simulink model "ex2"  (R2020a)
settings: Solver=VariableStepAuto  StartTime=0.0  StopTime=10.0  RelTol=1e-3
settings Model: Creator=EREN  LastModifiedBy=EREN

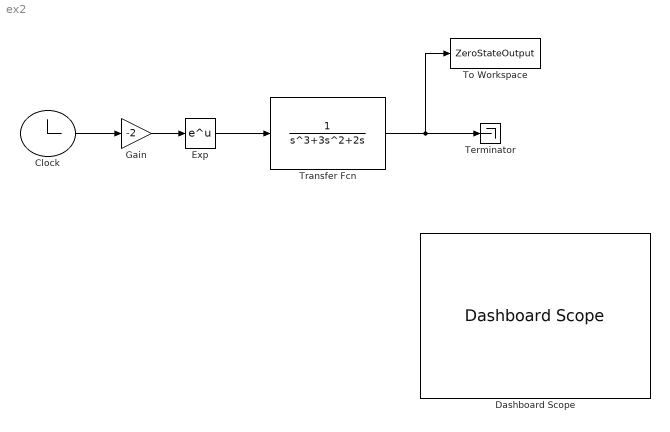
== system ex2 ==
  Clock : Clock
  Dashboard Scope : DashboardScope
  Exp : Math  SaturateOnIntegerOverflow=on
  Gain : Gain  Gain=-2
  Terminator : Terminator
  To Workspace : ToWorkspace  VariableName=ZeroStateOutput  SaveFormat=Timeseries  SampleTime=-1
  Transfer Fcn : TransferFcn  Denominator=[1 3 2 0]
  wires:
  Transfer Fcn/1 -> Terminator/1, To Workspace/1
  Exp/1 -> Transfer Fcn/1
  Clock/1 -> Gain/1
  Gain/1 -> Exp/1
